simulink model "gradfiltraspi"  (R2014b)
settings: Solver=FixedStepDiscrete  StartTime=0.0  StopTime=10.0  RelTol=1e-3
libraries: embdlinuxlib x2
settings Model: ExtModeTrigDuration=100  Creator=Shogo  LastModifiedBy=Shogo
settings OptimizationCC: OptimizeModelRefInitCode=on  LifeSpan=1
settings DebuggingCC: UnderspecifiedInitializationDetection=Classic  MergeDetectMultiDrivingBlocksExec=none  SolverPrmCheckMsg=none
settings HardwareCC: ProdLargestAtomicInteger=Long  ProdLargestAtomicFloat=Double  ProdEndianess=LittleEndian  ProdHWDeviceType=ARM Compatible->ARM Cortex
settings RTWCC: SystemTargetFile=realtime.tlc  GenerateMakefile=off  TemplateMakefile=realtime.tmf  Description=Run on Target Hardware  RTWVerbose=off  ProcessScript=realtime_make_rtw_hook
settings STFCustomTargetCC: TargetLibSuffix=.a  GenerateSampleERTMain=on  ERTCustomFileBanners=on  SupportNonInlinedSFcns=off  SupportVariableSizeSignals=on  MATLABClassNameForMDSCustomization=Simulink.SoftwareTarget.ERTCustomization  GRTInterface=off  SystemTargetFile=realtime.tlc
settings ERTTargetCC: GenerateSampleERTMain=on  ParMdlRefBuildCompliant=off  CompOptLevelCompliant=off  ConcurrentExecutionCompliant=off  CombineOutputUpdateFcns=off  ERTFirstTimeCompliant=off  SupportContinuousTime=on  SupportVariableSizeSignals=on  ModelStepFunctionPrototypeControlCompliant=off  CPPClassGenCompliant=off  ExtMode=on  ExtModeMexArgs='192.168.0.10' 0 17725 5  InlinedParameterPlacement=NonHierarchical  ERTSrcFileBannerTemplate=realtime_code_template.cgt  ERTHdrFileBannerTemplate=realtime_code_template.cgt  ERTDataSrcFileTemplate=realtime_code_template.cgt  ERTDataHdrFileTemplate=realtime_code_template.cgt  ERTCustomFileTemplate=realtime_file_process.tlc

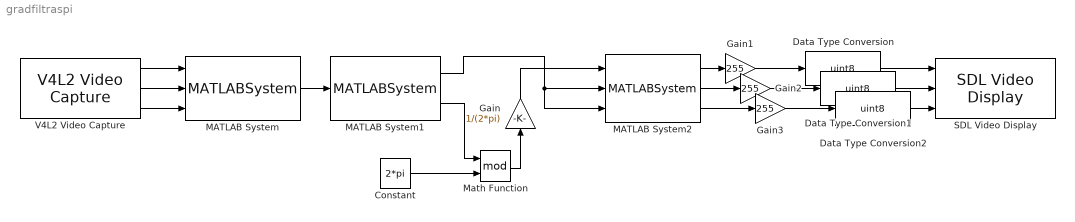
== system gradfiltraspi ==
  Constant : Constant  Value=2*pi  OutDataTypeStr=single
  Data Type Conversion : DataTypeConversion  OutDataTypeStr=uint8
  Data Type Conversion1 : DataTypeConversion  OutDataTypeStr=uint8
  Data Type Conversion2 : DataTypeConversion  OutDataTypeStr=uint8
  Gain : Gain  Gain=1/(2*pi)  OutDataTypeStr=single
  Gain1 : Gain  Gain=255
  Gain2 : Gain  Gain=255
  Gain3 : Gain  Gain=255
  MATLAB System : MATLABSystem  System=embvision.Rgb2GraySystem
      mask Type: embvision.Rgb2GraySystem
      mask Display:
      | disp('RGB2GRAY');
      | port_label('input',1,'R');
      | port_label('input',2,'G');
      | port_label('input',3,'B');
      | port_label('output',1,'Y');
  MATLAB System1 : MATLABSystem  System=embvision.GradFiltSystem  Kernel=[ 1, 0, -1; 1, 0, -1; 1, 0, -1 ].'
      mask Type: embvision.GradFiltSystem
      mask Display:
      | disp('GRAD_FILT');
      | port_label('input',1,'GRAY');
      | port_label('output',1,'MAG');
      | port_label('output',2,'ANG');
  MATLAB System2 : MATLABSystem  System=embvision.Hsv2RgbSystem
      mask Type: embvision.Hsv2RgbSystem
      mask Display:
      | disp('HSV2RGB');
      | port_label('input',1,'H');
      | port_label('input',2,'S');
      | port_label('input',3,'V');
      | port_label('output',1,'R');
      | port_label('output',2,'G');
      | port_label('output',3,'B');
  Math Function : Math  Operator=mod  OutputSignalType=real  SaturateOnIntegerOverflow=on
  SDL Video Display : embdlinuxlib/SDL Video Display  pixelFormat=RGB  pixelOrder=Planar  rowMajor=on  blockPlatform=Raspberry Pi
  V4L2 Video Capture : embdlinuxlib/V4L2 Video Capture  m_devName='/dev/video0'  roi=[0, 0, 640, 480]  imSizeSelection=160x120  imSize=[640, 480]  pixelFormat=RGB  pixelOrder=Planar  sampleTime=1/10  simOutput=Colorbars  blockPlatform=Raspberry Pi
  wires:
  V4L2 Video Capture/1 -> MATLAB System/1
  MATLAB System/1 -> MATLAB System1/1
  MATLAB System2/1 -> Gain1/1
  Gain/1 -> MATLAB System2/1
  MATLAB System1/1 -> MATLAB System2/3, MATLAB System2/2
  MATLAB System1/2 -> Math Function/1
  Math Function/1 -> Gain/1
  Constant/1 -> Math Function/2
  V4L2 Video Capture/2 -> MATLAB System/2
  V4L2 Video Capture/3 -> MATLAB System/3
  MATLAB System2/2 -> Gain2/1
  MATLAB System2/3 -> Gain3/1
  Data Type Conversion/1 -> SDL Video Display/1
  Data Type Conversion1/1 -> SDL Video Display/2
  Data Type Conversion2/1 -> SDL Video Display/3
  Gain1/1 -> Data Type Conversion/1
  Gain2/1 -> Data Type Conversion1/1
  Gain3/1 -> Data Type Conversion2/1
